simulink model "InverterFilter"  (R2022a)
settings: Solver=VariableStepAuto  StartTime=0.0  StopTime=0.1  RelTol=1e-3
libraries: spsIGBTDiodeLib x4, spsSeriesRLCBranchLib x4, simulink x2, spsCurrentMeasurementLib x2, spsVoltageMeasurementLib x2, spsDCVoltageSourceLib x1, spspowerguiLib x1
settings Model: Creator=nikke  LastModifiedBy=nikke

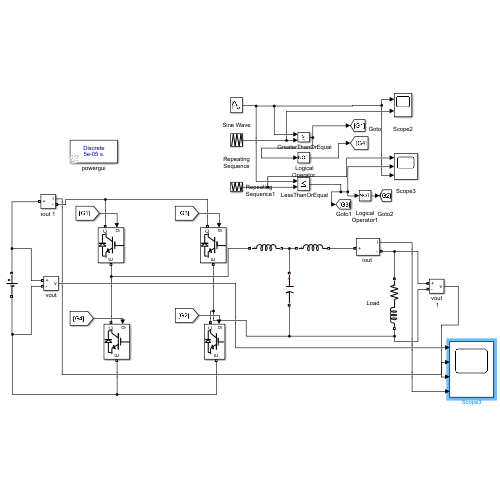
[thumbnail: Simulink's stored preview of the top-level diagram]
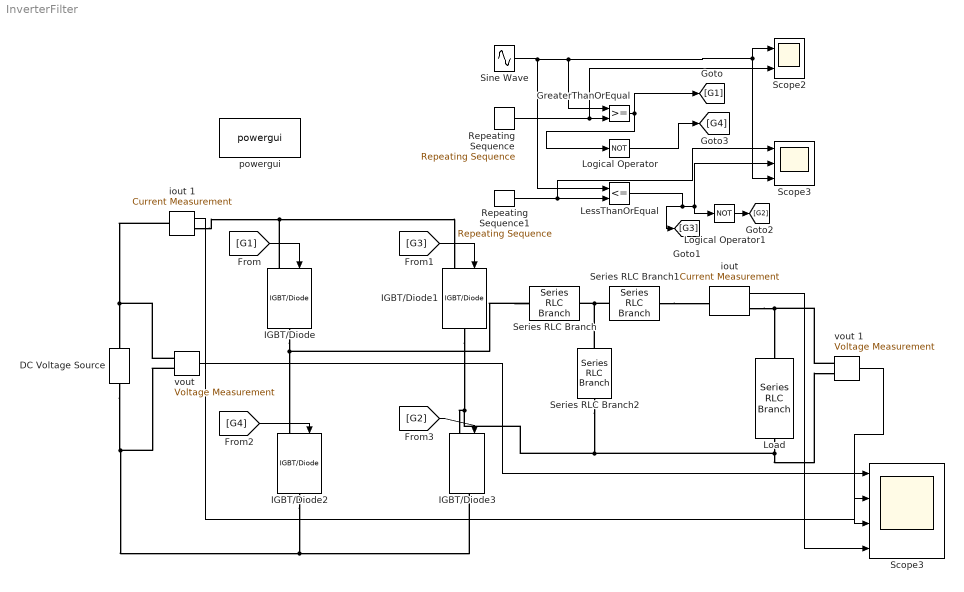
== system InverterFilter ==
  " Logical Operator1" : Logic  Operator=NOT  AllPortsSameDT=off  OutDataTypeStr=boolean
  " Repeating Sequence" : simulink/Sources/Repeating Sequence  rep_seq_t=[0 1/2 1]*(1/2000)  rep_seq_y=[0 1 0]
  " Repeating Sequence1" : simulink/Sources/Repeating Sequence  rep_seq_t=[0 1/2 1]*(1/1500)  rep_seq_y=[0 -1 0]
  " Scope3" : Scope  NumInputPorts=3
  " Sine Wave" : Sin  Amplitude=0.98  Frequency=2*pi*50  SampleTime=0
  " Scope2" : Scope  NumInputPorts=2
  " GreaterThanOrEqual" : RelationalOperator  OutDataTypeStr=boolean  RndMeth=Simplest  InputSameDT=off
  " LessThanOrEqual" : RelationalOperator  Operator=<=  OutDataTypeStr=boolean  RndMeth=Simplest  InputSameDT=off
  " Logical Operator" : Logic  Operator=NOT  AllPortsSameDT=off  OutDataTypeStr=boolean
  DC Voltage Source : spsDCVoltageSourceLib/DC Voltage Source  Amplitude=400  Measurements=None
  IGBT/Diode{,1..3} (4 alike) : spsIGBTDiodeLib/IGBT//Diode  Ron=1e-3  Rs=1e5  Cs=inf  Measurements=off
  Load : spsSeriesRLCBranchLib/Series RLC Branch  LConnTagsString=__new0  RConnTagsString=__new0  BranchType=RL  Resistance=27  Inductance=200e-3  SetiL0=off  InitialCurrent=0  Capacitance=100e-6  Setx0=off  InitialVoltage=0  Measurements=None
  Scope3 : Scope  NumInputPorts=4
  Series RLC Branch : spsSeriesRLCBranchLib/Series RLC Branch  LConnTagsString=__new0  RConnTagsString=__new0  BranchType=L  Resistance=1  Inductance=200e-3  SetiL0=off  InitialCurrent=0  Capacitance=1e-6  Setx0=off  InitialVoltage=0  Measurements=None
  Series RLC Branch1 : spsSeriesRLCBranchLib/Series RLC Branch  LConnTagsString=__new0  RConnTagsString=__new0  BranchType=L  Resistance=1  Inductance=200e-3  SetiL0=off  InitialCurrent=0  Capacitance=1e-6  Setx0=off  InitialVoltage=0  Measurements=None
  Series RLC Branch2 : spsSeriesRLCBranchLib/Series RLC Branch  LConnTagsString=__new0  RConnTagsString=__new0  BranchType=C  Resistance=1  Inductance=1e-3  SetiL0=off  InitialCurrent=0  Capacitance=18e-6  Setx0=off  InitialVoltage=0  Measurements=None
  "iout " : spsCurrentMeasurementLib/Current Measurement  PhasorSimulation=off  OutputType=Complex  PSBequivalent=0
  iout 1 : spsCurrentMeasurementLib/Current Measurement  PhasorSimulation=off  OutputType=Complex  PSBequivalent=0
  powergui : spspowerguiLib/powergui  Priority=1  SimulationMode=Discrete  SampleTime=50e-6  frequency=50  Iterations=50  frequencyindice=0  Pbase=100e6  ErrMax=1e-4  UnitsV=kV  UnitsW=MW  buscounter=0  FunctionMessages=off  echomessages=off  EnableUseOfTLC=off  CurrentSourceSwitches=off  DisableSnubberDevices=off  DisableRonSwitches=off  DisableVfSwitches=off  DisplayEquations=off  AutomaticDiscreteSolvers=off  SolverType=Tustin/Backward Euler (TBE)  Interpol=off  ExternalGateDelay=off  methode=off  Ts=100  x0status=blocks  SPID=on  SwTol=0  HookPort=off  NonlinearTolerance=1e-4  nMaxIteration=100  ContinueOnMaxIteration=off  RestoreLinks=warning  ResistiveCurrentMeasurement=off  Frange=[0:2:500]  Ylog=off  Xlog=on  ShowGrid=off  save=off  variable=ZData  structure=0  ZoomFFT=off  StartTime=0.0  cycles=1  DisplayStyle=1  fundamental=60  FreqAxis=off  MaxFrequency=1000  frequencyindicesteady=1  RmsSteady=1  display=off
  "vout " : spsVoltageMeasurementLib/Voltage Measurement  PhasorSimulation=off  OutputType=Complex  PSBequivalent=0
  vout 1 : spsVoltageMeasurementLib/Voltage Measurement  PhasorSimulation=off  OutputType=Complex  PSBequivalent=0
  wires:
  [G3] -> IGBT/Diode1/1
  [G2] -> IGBT/Diode3/1
  [G1] -> IGBT/Diode/1
  [G4] -> IGBT/Diode2/1
  " LessThanOrEqual"/1 -> " Logical Operator1"/1, " Scope3"/2, [G3]
  " Repeating Sequence1"/1 -> " LessThanOrEqual"/2, " Scope3"/1
  " Logical Operator1"/1 -> [G2]
  " Repeating Sequence"/1 -> " Scope2"/2, " GreaterThanOrEqual"/2
  " Logical Operator"/1 -> [G4]
  " Sine Wave"/1 -> " GreaterThanOrEqual"/1, " Scope3"/3, " Scope2"/1, " LessThanOrEqual"/1
  " GreaterThanOrEqual"/1 -> " Logical Operator"/1, [G1]
  "vout "/1 -> Scope3/1
  iout 1/1 -> Scope3/2
  vout 1/1 -> Scope3/3
  "iout "/1 -> Scope3/4
  connections:
  Series RLC Branch1/LConn1 -- Series RLC Branch2/LConn1 -- Series RLC Branch/RConn1
  Series RLC Branch1/RConn1 -- "iout "/LConn1
  IGBT/Diode/RConn1 -- Series RLC Branch/LConn1 -- IGBT/Diode2/LConn1
  vout 1/LConn1 -- "iout "/RConn1 -- Load/LConn1
  "vout "/LConn1 -- iout 1/LConn1 -- DC Voltage Source/RConn1
  IGBT/Diode3/RConn1 -- DC Voltage Source/LConn1 -- "vout "/LConn2 -- IGBT/Diode2/RConn1
  IGBT/Diode/LConn1 -- IGBT/Diode1/LConn1 -- iout 1/RConn1
  Load/RConn1 -- Series RLC Branch2/RConn1 -- IGBT/Diode1/RConn1 -- IGBT/Diode3/LConn1 -- vout 1/LConn2
